simulink model "Encoder_model"  (R2024b)
settings: Solver=FixedStepAuto  StartTime=0.0  StopTime=inf  FixedStep=0.01  RelTol=1e-3  EnableMultiTasking=on
model workspace (MAT data in the model file):
  x1_QEI_pos = 0
  x2_QEI_pos = 0
  x4_QEI_pos = 0
libraries: stm32f4xxblockslib x6, stm32g4xxblockslib x6, simulink x2
settings Model: STM32="{\"EncoderBlockForG4\":[{\"ID\":\"Encoder_model:2\"},{\"ID\":\"Encoder_model:75\"},{\"ID\":\"Encoder_model:82\"},{\"ID\":\"Encoder_model:107\"},{\"ID\":\"Encoder_model:108\"},{\"ID\":\"Encoder_model:109\"}],\"DigitalPortRead\":[{\"ID\":\"Encoder_model:14\"},{\"ID\":\"Encoder_model:15\"},{\"ID\":\"Encoder_model:129\"},{\"ID\":\"Encoder_model:131\"},{\"ID\":\"Encoder_model:116\"},{\"ID\":\"Encoder_model:117\"}]}"  Creator=jirat  LastModifiedBy=jirat
settings OptimizationCC: DefaultParameterBehavior=Inlined  EnhancedBackFolding=on  PassReuseOutputArgsAs=Individual arguments  ZeroExternalMemoryAtStartup=off  ZeroInternalMemoryAtStartup=off  MaxStackSize=512  OptimizeBlockOrder=speed  DifferentSizesBufferReuse=on  OptimizationCustomize=off  EfficientTunableParamExpr=on
settings DebuggingCC: ParameterTunabilityLossMsg=error
settings HardwareCC: ProdBitPerPointer=32  ProdBitPerSizeT=32  ProdBitPerPtrDiffT=32  ProdLargestAtomicInteger=Long  ProdLargestAtomicFloat=Double  ProdWordSize=32  ProdLongLongMode=on  ProdHWDeviceType=ARM Compatible->ARM Cortex-M
settings SFSimCC: MATLABDynamicMemAlloc=off
settings RTWCC: Description=Embedded Coder  SystemTargetFile=ert.tlc  HardwareBoard=STM32G4xx Based  TemplateMakefile=ert_default_tmf  Toolchain=GNU Tools for ARM Embedded Processors
settings CodeAppCC: ForceParamTrailComments=on  IgnoreCustomStorageClasses=off  OperatorAnnotations=on  SimulinkDataObjDesc=on  SFDataObjDesc=on  InsertBlockDesc=on
settings ERTTargetCC: TargetLangStandard=C99 (ISO)  CodeReplacementLibrary=ARM Cortex-M  ExtModeTransport=3  ExtModeStaticAlloc=on  ExtModeStaticAllocSize=2048  ExtModeMexFile=ext_xcp  ExtModeIntrfLevel=Level2 - Open

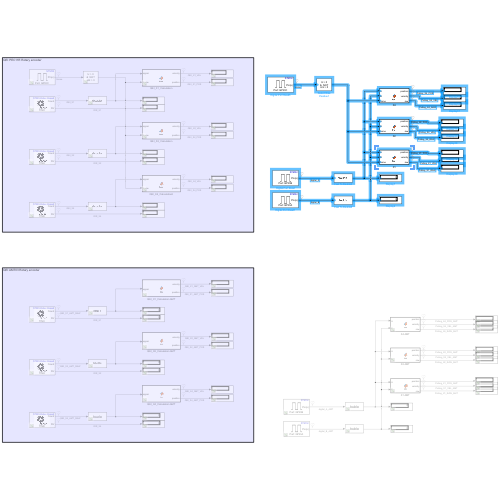
[thumbnail: Simulink's stored preview of the top-level diagram]
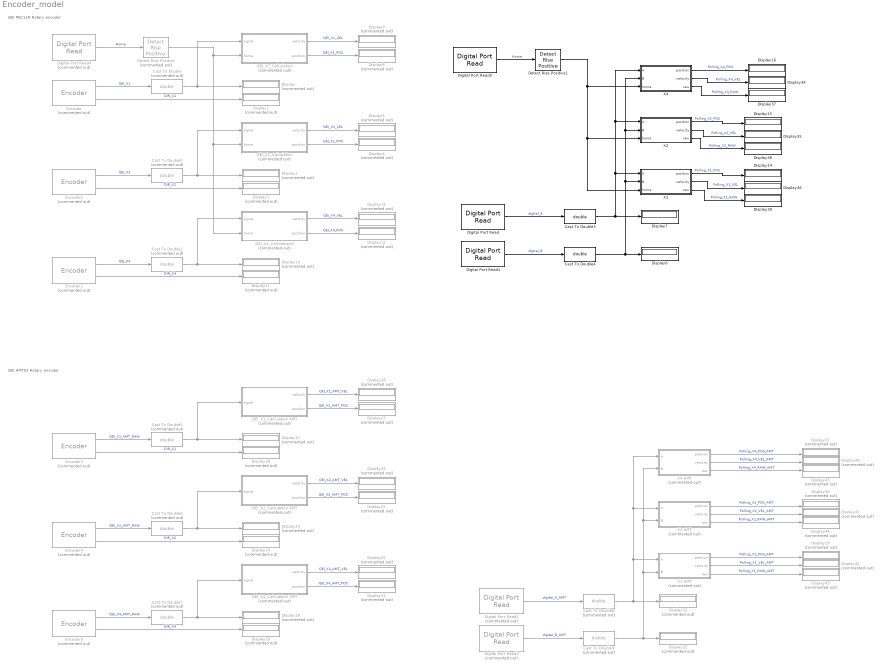
== system Encoder_model ==
  note: QEI PEC11R Rotary encoder
  note: QEI AMT03 Rotary encoder
  Cast To Double{,1..2,5..9} (8 alike) : DataTypeConversion  Commented=on  OutDataTypeStr=double  SaturateOnIntegerOverflow=off  RndMeth=Floor
  Cast To Double3 : DataTypeConversion  OutDataTypeStr=double  SaturateOnIntegerOverflow=off  RndMeth=Floor
  Cast To Double4 : DataTypeConversion  OutDataTypeStr=double  SaturateOnIntegerOverflow=off  RndMeth=Floor
  Detect Rise Positive : simulink/Logic and Bit Operations/Detect Rise Positive  Commented=on  vinit=0  OutDataTypeStr=boolean
  Detect Rise Positive1 : simulink/Logic and Bit Operations/Detect Rise Positive  vinit=0  OutDataTypeStr=boolean
  Digital Port Read : stm32f4xxblockslib/Digital Port Read  PortName=GPIOB  PinNumber=[5]  ReadOperation=on  IOAsArray=on  SampleTime=-1  EnableSimPort=off  hoistedMaskSrc=ECSoC/ECSimCodegen/Digital Port Read
      settings: LibrarySourceBlock=stm32g4xxblockslib/Digital Port Read
  Digital Port Read1 : stm32f4xxblockslib/Digital Port Read  PortName=GPIOA  PinNumber=[10]  ReadOperation=on  IOAsArray=on  SampleTime=-1  EnableSimPort=off  hoistedMaskSrc=ECSoC/ECSimCodegen/Digital Port Read
      settings: LibrarySourceBlock=stm32g4xxblockslib/Digital Port Read
  Digital Port Read2 : stm32f4xxblockslib/Digital Port Read  Commented=on  PortName=GPIOB  PinNumber=[5]  ReadOperation=on  IOAsArray=on  SampleTime=-1  EnableSimPort=off  hoistedMaskSrc=ECSoC/ECSimCodegen/Digital Port Read
      settings: LibrarySourceBlock=stm32g4xxblockslib/Digital Port Read
  Digital Port Read3 : stm32f4xxblockslib/Digital Port Read  Commented=on  PortName=GPIOA  PinNumber=[10]  ReadOperation=on  IOAsArray=on  SampleTime=-1  EnableSimPort=off  hoistedMaskSrc=ECSoC/ECSimCodegen/Digital Port Read
      settings: LibrarySourceBlock=stm32g4xxblockslib/Digital Port Read
  Digital Port Read4 : stm32f4xxblockslib/Digital Port Read  Commented=on  PortName=GPIOC  PinNumber=[13]  ReadOperation=on  IOAsArray=on  SampleTime=-1  EnableSimPort=off  hoistedMaskSrc=ECSoC/ECSimCodegen/Digital Port Read
      settings: LibrarySourceBlock=stm32g4xxblockslib/Digital Port Read
  Digital Port Read5 : stm32f4xxblockslib/Digital Port Read  PortName=GPIOC  PinNumber=[13]  ReadOperation=on  IOAsArray=on  SampleTime=-1  EnableSimPort=off  hoistedMaskSrc=ECSoC/ECSimCodegen/Digital Port Read
      settings: LibrarySourceBlock=stm32g4xxblockslib/Digital Port Read
  Display{,1..5,8..13,17..33,40..45} (35 alike) : Display  Commented=on
  Display{6..7,14..16,34..39} (11 alike) : Display
  Encoder : stm32g4xxblockslib/Encoder  Commented=on  TimerModule=TIM3  EnableResetInput=off  OutputCountAfterFirstIndex=off  OutputValidIndex=off  OutputDirection=on  OutputStatus=off  SampleTime=-1
  Encoder1 : stm32g4xxblockslib/Encoder  Commented=on  TimerModule=TIM4  EnableResetInput=off  OutputCountAfterFirstIndex=off  OutputValidIndex=off  OutputDirection=on  OutputStatus=off  SampleTime=-1
  Encoder2 : stm32g4xxblockslib/Encoder  Commented=on  TimerModule=TIM8  EnableResetInput=off  OutputCountAfterFirstIndex=off  OutputValidIndex=off  OutputDirection=on  OutputStatus=off  SampleTime=-1
  Encoder3 : stm32g4xxblockslib/Encoder  Commented=on  TimerModule=TIM3  EnableResetInput=off  OutputCountAfterFirstIndex=off  OutputValidIndex=off  OutputDirection=on  OutputStatus=off  SampleTime=-1
  Encoder4 : stm32g4xxblockslib/Encoder  Commented=on  TimerModule=TIM4  EnableResetInput=off  OutputCountAfterFirstIndex=off  OutputValidIndex=off  OutputDirection=on  OutputStatus=off  SampleTime=-1
  Encoder5 : stm32g4xxblockslib/Encoder  Commented=on  TimerModule=TIM8  EnableResetInput=off  OutputCountAfterFirstIndex=off  OutputValidIndex=off  OutputDirection=on  OutputStatus=off  SampleTime=-1
  QEI_X1_Calculation : MATLAB Function  Commented=on  TreatAsAtomicUnit=on
  QEI_X1_Calculation AMT : MATLAB Function  Commented=on  TreatAsAtomicUnit=on
  QEI_X2_Calculation : MATLAB Function  Commented=on  TreatAsAtomicUnit=on
  QEI_X2_Calculation AMT : MATLAB Function  Commented=on  TreatAsAtomicUnit=on
  QEI_X4_Calculation AMT : MATLAB Function  Commented=on  TreatAsAtomicUnit=on
  QEI_X4_Calculation2 : MATLAB Function  Commented=on  TreatAsAtomicUnit=on
  X1 : MATLAB Function  TreatAsAtomicUnit=on
  X1 AMT : MATLAB Function  Commented=on  TreatAsAtomicUnit=on
  X2 : MATLAB Function  TreatAsAtomicUnit=on
  X2 AMT : MATLAB Function  Commented=on  TreatAsAtomicUnit=on
  X4 : MATLAB Function  TreatAsAtomicUnit=on
  X4 AMT : MATLAB Function  Commented=on  TreatAsAtomicUnit=on
  wires:
  Encoder/1 -> Cast To Double/1  "QEI_X1"
  Cast To Double/1 -> QEI_X1_Calculation/1(signal), Display/1
  Encoder/2 -> Display1/1  "DIR_X1"
  Digital Port Read1/1 -> Cast To Double4/1  "digital_B"
  Digital Port Read/1 -> Cast To Double3/1  "digital_A"
  QEI_X1_Calculation/2(position) -> Display8/1  "QEI_X1_POS"
  QEI_X1_Calculation/1(velocity) -> Display9/1  "QEI_X1_VEL"
  QEI_X2_Calculation/1(velocity) -> Display5/1  "QEI_X2_VEL"
  Cast To Double1/1 -> QEI_X2_Calculation/1(signal), Display2/1
  Encoder1/1 -> Cast To Double1/1  "QEI_X2"
  Encoder1/2 -> Display3/1  "DIR_X2"
  QEI_X2_Calculation/2(position) -> Display4/1  "QEI_X2_POS"
  QEI_X4_Calculation2/1(velocity) -> Display13/1  "QEI_X4_VEL"
  Cast To Double2/1 -> QEI_X4_Calculation2/1(signal), Display10/1
  Encoder2/1 -> Cast To Double2/1  "QEI_X4"
  Encoder2/2 -> Display11/1  "DIR_X4"
  QEI_X4_Calculation2/2(position) -> Display12/1  "QEI_X4_POS"
  X1/1(position) -> Display14/1  "Polling_X1_POS"
  X2/1(position) -> Display15/1  "Polling_X2_POS"
  Cast To Double4/1 -> X4/2(B), X2/2(B), X1/2(B), Display6/1
  Cast To Double3/1 -> X4/1(A), X2/1(A), X1/1(A), Display7/1
  X4/1(position) -> Display16/1  "Polling_X4_POS"
  QEI_X4_Calculation AMT/1(velocity) -> Display22/1  "QEI_X4_AMT_VEL"
  Cast To Double6/1 -> QEI_X2_Calculation AMT/1(signal), Display23/1
  QEI_X2_Calculation AMT/1(velocity) -> Display26/1  "QEI_X2_AMT_VEL"
  QEI_X4_Calculation AMT/2(position) -> Display21/1  "QEI_X4_AMT_POS"
  Cast To Double7/1 -> QEI_X4_Calculation AMT/1(signal), Display19/1
  Encoder5/1 -> Cast To Double7/1  "QEI_X4_AMT_RAW"
  Encoder4/2 -> Display24/1  "DIR_X2"
  Encoder4/1 -> Cast To Double6/1  "QEI_X2_AMT_RAW"
  Cast To Double5/1 -> QEI_X1_Calculation AMT/1(signal), Display17/1
  Encoder3/1 -> Cast To Double5/1  "QEI_X1_AMT_RAW"
  QEI_X2_Calculation AMT/2(position) -> Display25/1  "QEI_X2_AMT_POS"
  QEI_X1_Calculation AMT/2(position) -> Display27/1  "QEI_X1_AMT_POS"
  Encoder3/2 -> Display18/1  "DIR_X1"
  QEI_X1_Calculation AMT/1(velocity) -> Display28/1  "QEI_X1_AMT_VEL"
  Encoder5/2 -> Display20/1  "DIR_X4"
  Cast To Double8/1 -> X4 AMT/1(A), X2 AMT/1(A), X1 AMT/1(A), Display33/1
  Digital Port Read3/1 -> Cast To Double9/1  "digital_B_AMT"
  Cast To Double9/1 -> X4 AMT/2(B), X2 AMT/2(B), X1 AMT/2(B), Display32/1
  X1 AMT/1(position) -> Display29/1  "Polling_X1_POS_AMT"
  X2 AMT/1(position) -> Display30/1  "Polling_X2_POS_AMT"
  Digital Port Read2/1 -> Cast To Double8/1  "digital_A_AMT"
  X4 AMT/1(position) -> Display31/1  "Polling_X4_POS_AMT"
  X4/2(velocity) -> Display34/1  "Polling_X4_VEL"
  X2/2(velocity) -> Display35/1  "Polling_X2_VEL"
  X1/2(velocity) -> Display36/1  "Polling_X1_VEL"
  Digital Port Read4/1 -> Detect Rise Positive/1  "Home"
  Detect Rise Positive/1 -> QEI_X4_Calculation2/2(home), QEI_X2_Calculation/2(home), QEI_X1_Calculation/2(home)
  Digital Port Read5/1 -> Detect Rise Positive1/1  "Home"
  Detect Rise Positive1/1 -> X1/3(home), X2/3(home), X4/3(home)
  X4/3(raw) -> Display37/1  "Polling_X4_RAW"
  X2/3(raw) -> Display38/1  "Polling_X2_RAW"
  X1/3(raw) -> Display39/1  "Polling_X1_RAW"
  X4 AMT/2(velocity) -> Display40/1  "Polling_X4_VEL_AMT"
  X2 AMT/2(velocity) -> Display41/1  "Polling_X2_VEL_AMT"
  X1 AMT/2(velocity) -> Display42/1  "Polling_X1_VEL_AMT"
  X4 AMT/3(raw) -> Display43/1  "Polling_X4_RAW_AMT"
  X2 AMT/3(raw) -> Display44/1  "Polling_X2_RAW_AMT"
  X1 AMT/3(raw) -> Display45/1  "Polling_X1_RAW_AMT"

== matlab function Encoder_model/X2 AMT ==
  data: A input; position output; B input; velocity output; raw output
function [position,velocity,raw] = fcn(A,B)

persistent pre_A
persistent pre_B

if isempty(pre_A)
    pre_A = 1;
end
if isempty(pre_B)
    pre_B = 1;
end

persistent pos;
persistent pre_pos;
persistent vel;
if isempty(pos)
    pos = 0;
end
if isempty(pre_pos)
    pre_pos = 0;
end
if isempty(vel)
    vel = 0;
end

if A == 0 && pre_A == 1
    if B == 1
        pos = pos + 1;
    else 
        pos = pos - 1;
    end
end

if A == 1 && pre_A == 0
    if B == 0
        pos = pos + 1;
    else
        pos = pos - 1;
    end
end

% Velocity Calculation 
delta_P = pos - pre_pos;
vel = delta_P / 0.01;
vel = (vel/4096) * (2*pi);
   
velocity = vel;
position = (pos * 1/4096 * 2 * pi);
raw = pos;
pre_pos = pos;
pre_A = A;
pre_B = B;

== matlab function Encoder_model/QEI_X2_Calculation ==
  data: signal input; velocity output; position output; home input
function [velocity,position]= fcn(signal,home)

% Previous data configuration
persistent pos;
persistent pre_signal;
persistent vel;
persistent array_pos;
if isempty(array_pos)
    array_pos = zeros(1,10);
end
if isempty(pos)
    pos = 0;
end
if isempty(pre_signal)
    pre_signal = 0;
end
if isempty(vel)
    vel = 0;
end

diff = signal - pre_signal;

% Homing
if home == 1
    pos = 0;
    array_pos = zeros(1,10);
end

% Position calculation
if diff < -65472/2
    pos = pos + (signal + (65473 - pre_signal));
    
elseif diff > 65472/2
    pos = pos - (pre_signal + (65473 - signal));
else
    pos = pos + diff;
end

% Moving array
array_pos = [pos,array_pos(1:end-1)];

% Velocity Calculation 
delta_P = array_pos(1) - array_pos(10);
vel = delta_P / 0.1;
vel = (vel/48) * (2*pi);

% Return data
position = (pos * 1/48 * 2 * pi);
velocity = vel;
% Clean previous data
pre_signal = signal;
% pre_pos = pos;

== matlab function Encoder_model/X4 AMT ==
  data: A input; position output; B input; velocity output; raw output
function [position,velocity,raw] = fcn(A,B)

persistent pre_A
persistent pre_B

if isempty(pre_A)
    pre_A = 1;
end
if isempty(pre_B)
    pre_B = 1;
end

persistent pos;
persistent pre_pos;
persistent vel;
if isempty(pos)
    pos = 0;
end
if isempty(pre_pos)
    pre_pos = 0;
end
if isempty(vel)
    vel = 0;
end

if A == 0 && pre_A == 1
    if B == 1
        pos = pos + 1;
    else 
        pos = pos - 1;
    end
end

if A == 1 && pre_A == 0
    if B == 0
        pos = pos + 1;
    else
        pos = pos - 1;
    end
end
if B == 0 && pre_B == 1
    if A == 0
        pos = pos + 1;
    else
        pos = pos - 1;
    end
end

if B == 1 && pre_B == 0
    if A == 1
        pos = pos + 1;
    else
        pos = pos - 1;
    end
end

% Velocity Calculation 
delta_P = pos - pre_pos;
vel = delta_P / 0.01;
vel = (vel/8192) * (2*pi);

velocity = vel;
position = (pos * 1/8192 * 2 * pi);
raw = pos;
pre_pos = pos;
pre_A = A;
pre_B = B;

== matlab function Encoder_model/QEI_X1_Calculation ==
  data: signal input; velocity output; position output; home input
function [velocity,position]= fcn(signal,home)

% Previous data configuration
persistent pos;
persistent pre_signal;
persistent vel;
persistent array_pos;
if isempty(array_pos)
    array_pos = zeros(1,10);
end
if isempty(pos)
    pos = 0;
end
if isempty(pre_signal)
    pre_signal = 0;
end
if isempty(vel)
    vel = 0;
end

diff = signal - pre_signal;

% Homing
if home == 1
    pos = 0;
    array_pos = zeros(1,10);
end

% Position calculation
if diff < -65472/2
    pos = pos + (signal + (65473 - pre_signal));
elseif diff > 65472/2
    pos = pos - (pre_signal + (65473 - signal));
else
    pos = pos + diff;
end

% Moving array
array_pos = [pos,array_pos(1:end-1)];

% Velocity Calculation 
delta_P = array_pos(1) - array_pos(10);
vel = delta_P / 0.1;
vel = (vel/24) * (2*pi);

% Return data
position = (pos * 1/24 * 2 * pi);
velocity = vel;
% Clean previous data
pre_signal = signal;
% pre_pos = pos;

== matlab function Encoder_model/QEI_X4_Calculation2 ==
  data: signal input; velocity output; position output; home input
function [velocity,position]= fcn(signal,home)

% Previous data configuration
persistent pos;
persistent pre_signal;
persistent vel;
persistent array_pos;
if isempty(array_pos)
    array_pos = zeros(1,10);
end
if isempty(pos)
    pos = 0;
end
if isempty(pre_signal)
    pre_signal = 0;
end
if isempty(vel)
    vel = 0;
end

diff = signal - pre_signal;

% Homing
if home == 1
    pos = 0;
    array_pos = zeros(1,10);
end

% Position calculation
if diff < -65472/2
    pos = pos + (signal + (65473 - pre_signal));
    
elseif diff > 65472/2
    pos = pos - (pre_signal + (65473 - signal));
else
    pos = pos + diff;
end

% Moving array
array_pos = [pos,array_pos(1:end-1)];

% Velocity Calculation 
delta_P = array_pos(1) - array_pos(10);
vel = delta_P / 0.1;
vel = (vel/96) * (2*pi);

% Return data
position = (pos * 1/96 * 2 * pi);
velocity = vel;
% Clean previous data
pre_signal = signal;
% pre_pos = pos;

== matlab function Encoder_model/X1 ==
  data: A input; position output; B input; velocity output; home input; raw output
function [position,velocity,raw] = fcn(A,B,home)

persistent pre_A
persistent pre_B

if isempty(pre_A)
    pre_A = 1;
end
if isempty(pre_B)
    pre_B = 1;
end

persistent pos;
persistent array_pos;
if isempty(array_pos)
    array_pos = zeros(1,10);
end
persistent vel;
if isempty(pos)
    pos = 0;
end
if isempty(vel)
    vel = 0;
end

% Homing
if home == 1
    pos = 0;
    array_pos = zeros(1,10);
end

% Pos measure X1
if A == 0 && pre_A == 1
    if B == 1
        pos = pos + 1;
    else 
        pos = pos - 1;
    end
end

% Moving array
array_pos = [pos,array_pos(1:end-1)];

% Velocity Calculation 
delta_P = array_pos(1) - array_pos(10);
vel = delta_P / 0.1;
vel = (vel/24) * (2*pi);
   
velocity = vel;
raw = pos;
position = (pos * 1/24 * 2 * pi);
pre_A = A;
pre_B = B;

== matlab function Encoder_model/X2 ==
  data: A input; position output; B input; velocity output; home input; raw output
function [position,velocity,raw] = fcn(A,B,home)

persistent pre_A
persistent pre_B

if isempty(pre_A)
    pre_A = 1;
end
if isempty(pre_B)
    pre_B = 1;
end

persistent pos;
persistent array_pos;
if isempty(array_pos)
    array_pos = zeros(1,10);
end
persistent vel;
if isempty(pos)
    pos = 0;
end
if isempty(vel)
    vel = 0;
end

% Homing
if home == 1
    pos = 0;
    array_pos = zeros(1,10);
end

% Pos measure X2
if A == 0 && pre_A == 1
    if B == 1
        pos = pos + 1;
    else 
        pos = pos - 1;
    end
end

if A == 1 && pre_A == 0
    if B == 0
        pos = pos + 1;
    else
        pos = pos - 1;
    end
end
   
% Moving array
array_pos = [pos,array_pos(1:end-1)];

% Velocity Calculation 
delta_P = array_pos(1) - array_pos(10);
vel = delta_P / 0.1;
vel = (vel/48) * (2*pi);
   
velocity = vel;
raw = pos;
position = (pos * 1/48 * 2 * pi);
pre_A = A;
pre_B = B;

== matlab function Encoder_model/X4 ==
  data: A input; position output; B input; velocity output; home input; raw output
function [position,velocity,raw] = fcn(A,B, home)

persistent pre_A
persistent pre_B

if isempty(pre_A)
    pre_A = 1;
end
if isempty(pre_B)
    pre_B = 1;
end

persistent pos;
persistent array_pos;
if isempty(array_pos)
    array_pos = zeros(1,10);
end
persistent vel;
if isempty(pos)
    pos = 0;
end
if isempty(vel)
    vel = 0;
end

% Homing
if home == 1
    pos = 0;
    array_pos = zeros(1,10);
end

% Pos measure X4
if A == 0 && pre_A == 1
    if B == 1
        pos = pos + 1;
    else 
        pos = pos - 1;
    end
end

if A == 1 && pre_A == 0
    if B == 0
        pos = pos + 1;
    else
        pos = pos - 1;
    end
end
if B == 0 && pre_B == 1
    if A == 0
        pos = pos + 1;
    else
        pos = pos - 1;
    end
end

if B == 1 && pre_B == 0
    if A == 1
        pos = pos + 1;
    else
        pos = pos - 1;
    end
end

% Moving array
array_pos = [pos,array_pos(1:end-1)];

% Velocity Calculation 
delta_P = array_pos(1) - array_pos(10);
vel = delta_P / 0.1;
vel = (vel/96) * (2*pi);
   
velocity = vel;
raw = pos;
position = (pos * 1/96 * 2 * pi);
pre_A = A;
pre_B = B;

== matlab function Encoder_model/QEI_X1_Calculation AMT ==
  data: signal input; velocity output; position output
function [velocity,position]= fcn(signal)

% Previous data configuration
persistent pos;
persistent pre_signal;
persistent vel;
persistent pre_pos;
if isempty(pre_pos)
    pre_pos = 0;
end
if isempty(pos)
    pos = 0;
end
if isempty(pre_signal)
    pre_signal = 0;
end
if isempty(vel)
    vel = 0;
end

diff = signal - pre_signal;

% Position calculation
if diff < -57344/2
    pos = pos + (signal + (57345 - pre_signal));
    
elseif diff > 57344/2
    pos = pos - (pre_signal + (57345 - signal));
else
    pos = pos + diff;
end

% Velocity Calculation 
delta_P = pos - pre_pos;
vel = delta_P / 0.01;
vel = (vel/2048) * (2*pi);

% Return data
position = (pos * 1/2048 * 2 * pi);
% position = pos;
velocity = vel;
% Clean previous data
pre_signal = signal;
pre_pos = pos;

== matlab function Encoder_model/QEI_X2_Calculation AMT ==
  data: signal input; velocity output; position output
function [velocity,position]= fcn(signal)

% Previous data configuration
persistent pos;
persistent pre_signal;
persistent vel;
persistent pre_pos;
if isempty(pre_pos)
    pre_pos = 0;
end
if isempty(pos)
    pos = 0;
end
if isempty(pre_signal)
    pre_signal = 0;
end
if isempty(vel)
    vel = 0;
end

diff = signal - pre_signal;

% Position calculation
if diff < -57344/2
    pos = pos + (signal + (57345 - pre_signal));
    
elseif diff > 57344/2
    pos = pos - (pre_signal + (57345 - signal));
else
    pos = pos + diff;
end

% Velocity Calculation 
delta_P = pos - pre_pos;
vel = delta_P / 0.01;
vel = (vel/4096) * (2*pi);

% Return data
 position = (pos * 1/4096 * 2 * pi);
% position = pos;
velocity = vel;
% Clean previous data
pre_signal = signal;
pre_pos = pos;

== matlab function Encoder_model/QEI_X4_Calculation AMT ==
  data: signal input; velocity output; position output
function [velocity,position]= fcn(signal)

% Previous data configuration
persistent pos;
persistent pre_signal;
persistent vel;
persistent pre_pos;
if isempty(pre_pos)
    pre_pos = 0;
end
if isempty(pos)
    pos = 0;
end
if isempty(pre_signal)
    pre_signal = 0;
end
if isempty(vel)
    vel = 0;
end

diff = signal - pre_signal;

% Position calculation
if diff < -57344/2
    pos = pos + (signal + (57345 - pre_signal));
    
elseif diff > 57344/2
    pos = pos - (pre_signal + (57345 - signal));
else
    pos = pos + diff;
end

% Velocity Calculation 
delta_P = pos - pre_pos;
vel = delta_P / 0.01;
vel = (vel/8192) * (2*pi);

% Return data
position = (pos * 1/8192 * 2 * pi);
% position = pos;
velocity = vel;
% Clean previous data
pre_signal = signal;
pre_pos = pos;

== matlab function Encoder_model/X1 AMT ==
  data: A input; position output; B input; velocity output; raw output
function [position,velocity, raw] = fcn(A,B)

persistent pre_A
persistent pre_B

if isempty(pre_A)
    pre_A = 1;
end
if isempty(pre_B)
    pre_B = 1;
end

persistent pos;
persistent pre_pos;
persistent vel;
if isempty(pos)
    pos = 0;
end
if isempty(pre_pos)
    pre_pos = 0;
end
if isempty(vel)
    vel = 0;
end

if A == 0 && pre_A == 1
    if B == 1
        pos = pos + 1;
    else 
        pos = pos - 1;
    end
end

% Velocity Calculation 
delta_P = pos - pre_pos;
vel = delta_P / 0.01;
vel = (vel/2048) * (2*pi);
   
velocity = vel;
position = (pos * 1/2048 * 2 * pi);
raw = pos;
pre_pos = pos;
pre_A = A;
pre_B = B;
